simulink model "MSDRPrimaryLoop_LoadFollow"  (R2021b)
settings: Solver=VariableStepAuto  StartTime=0.0  StopTime=604900  MaxStep=1  MinStep=0.01  RelTol=1e-3
undefined symbols (not defined in the file): a_f, A_free_PHX, a_g, A_h_PHX, beta, beta_t, bubbleGeneratorArea, bubbleGeneratorDh, bubbleGeneratorElevation, bubbleGeneratorLength, bubbleGeneratorVolume, bubbleSaturationLevel, bubbleSeparatorArea, bubbleSeparatorDiameter, bubbleSeparatorDo, bubbleSeparatorLength, bubbleSeparatorSlope, bypassRatio, C0, coreFlowArea, coreFuelVolume, coreLowerPlenumArea, coreLowerPlenumHydraulicDiameter, coreLowerPlenumLength, coreLowerPlenumVolume, coreUpperPlenumArea, coreUpperPlenumHydraulicDiameter, coreUpperPlenumLength, coreUpperPlenumVolume, coreVolume, cpGraphite, dissolusionRatio, dMin, dScale, dsmConst, DXeG, Fiss_factor, fuelChannelHydrualicDiameter, fuelChannelLength, fuelDepositRatio, fuelFraction, fuelGraphiteArea, fuelGraphiteHeatTransferCoefficient, gamma0, gamma1, gamma2, generatorDsm, graphiteKDiff, graphiteUnitCellThickness, initialIodineConcentration, InitialXeMolarConcentration, InjectionRatio, injectionRatio, iodineDecayConstant, IodineDecayConstant, iodineYield, kGraphite, kScale, Lam, lam ... (+60)
libraries: fl_lib x268, nesl_utility x106, SimscapeFluids_lib x20, slpidlib x1
(part 12 of 12)

== system MSDRPrimaryLoop_LoadFollow/Reactor/CoreTH&Inerti/Core/CoreXenonCalc/InterphaseTranfser/Constitutive ==
  alpha : Inport
  PLoss : Inport  Port=2
  VolumeRate : Inport  Port=3
  Diam : Inport  Port=4
  Absolute Reference (TL) : fl_lib/Thermal Liquid/Elements/Absolute Reference (TL)
      settings: SourceProductBaseCode=SS
  DiffusivityScale : Subsystem  ReferencedSubsystem=DiffusivityScale
  Divide : Product  Inputs=**/
  Divide1 : Product  Inputs=*/
  KScale : Subsystem  ReferencedSubsystem=KScale
  PS-Simulink Converter : nesl_utility/PS-Simulink Converter  PhysicalDomain=network_engine_domain  SubClassName=ps_output  LeftPortType=input  RightPortType=output  PseudoPeriodic=off  Frequencies=[]  Unit=inherit  AffineConversion=off
      settings: SourceProductBaseCode=PW,SS
  PS-Simulink Converter2 : nesl_utility/PS-Simulink Converter  PhysicalDomain=network_engine_domain  SubClassName=ps_output  LeftPortType=input  RightPortType=output  PseudoPeriodic=off  Frequencies=[]  Unit=inherit  AffineConversion=off
      settings: SourceProductBaseCode=PW,SS
  Pressure & Temperature Sensor (TL) : fl_lib/Thermal Liquid/Sensors/Pressure & Temperature Sensor (TL)
      settings: SourceProductBaseCode=SS  InternalSimscapePortConfiguration="{\"Bottom\":[],\"Left\":[{\"id\":\"A\",\"label\":\"A\",\"type\":\"foundation.thermal_liquid.thermal_liquid\"}],\"Right\":[{\"id\":\"B\",\"label\":\"B\",\"type\":\"foundation.thermal_liquid.thermal_liquid\"},{\"id\":\"P\",\"label\":\"P\",\"type\":\"output\"},{\"id\":\"T\",\"label\":\"T\",\"type\":\"output\"}],\"Top\":[]}"
  RateToVelocity : Gain  Gain=1/CoreFlowArea
  Simscape Component : SimscapeComponentBlock  SourceFile=TL_FullSensor  ComponentPath=TL_FullSensor  ComponentVariants="[\"TL_FullSensor\"]"  ComponentVariantNames="[\"TL_FullSensor\"]"  ClassName=TL_FullSensor  SchemaVersion=1
      settings: CopyFcn=simscape.engine.sli.internal.componentblockcallback(gcbh,'COPY')  PreCopyFcn=simscape.engine.sli.internal.componentblockcallback(gcbh,'PRECOPY')  PreDeleteFcn=simscape.engine.sli.internal.componentblockcallback(gcbh,'PREDELETE')  InternalSimscapePortConfiguration="{\"Bottom\":[],\"Left\":[{\"id\":\"A\",\"label\":\"A\",\"type\":\"foundation.thermal_liquid.thermal_liquid\"}],\"Right\":[{\"id\":\"U\",\"label\":\"u\",\"type\":\"output\"},{\"id\":\"RHO\",\"label\":\"rho\",\"type\":\"output\"},{\"id\":\"CP\",\"label\":\"cp\",\"type\":\"output\"},{\"id\":\"NU\",\"label\":\"nu\",\"type\":\"output\"}],\"Top\":[]}"
      mask Type: Thermodynamic Properties Sensor (TL)
  Subsystem : Subsystem
      settings: PortSchema="{\"entries\":[{\"content\":{\"sides\":[{\"content\":{\"connectorIds\":[\"In1\",\"In2\",\"In3\"]},\"type\":\"ConnectorPlacement.EquallySpacedRectSide\",\"uuid\":\"97ac891d-0429-4bc8-a60c-b0f3d1709d12\"},{\"content\":{\"connectorIds\":[\"Out1\",\"Out2\"],\"side\":\"RIGHT\"},\"type\":\"ConnectorPlacement.EquallySpacedRectSide\",\"uuid\":\"927322a9-25fd-4042-b3db-749c2dfc8e8e\"},{\"content\":{\"connectorIds\":[\"In4\"],\"side\":\"TOP\"},\"type\":\"ConnectorPlacement.EquallySpacedRectSide\",\"uuid\":\"5b5a100b-866f-4829-ad8d-b4d6b97554c9\"},{\"content\":{\"connectorIds\":[\"RConn1\"],\"side\":\"BOTTOM\"},\"type\":\"ConnectorPlacement.EquallySpacedRectSide\",\"uuid\":\"36595118-997d-4e8e-8858-46ba20a030b3\"}]},\"type\":\"ConnectorPlacement.EquallySpacedConnector\",\"uuid\":\"6add3457-58ee-40cf-aa0f-ff6fc47a0098\"}],\"packageUris\":[\"http://schema.mathworks.com/mf0/Connector/R2020b\"],\"version\":\"1.0\"}"
  Ref : PMIOPort  Side=Left
  ul : Outport
  ug : Outport  Port=2
  K : Outport  Port=3
  Re : Outport  Port=4
  Sc : Outport  Port=5
  Diff : Outport  Port=6
  alphaC : Outport  Port=7
  dsm : Outport  Port=8
  f_m : Outport  Port=9
  wires:
  alpha/1 -> alphaC/1, Subsystem/4(alpha)
  VolumeRate/1 -> RateToVelocity/1
  RateToVelocity/1 -> ug/1, Subsystem/3(ul), ul/1, Divide/1
  Diam/1 -> Subsystem/2(Dh), Divide/2
  PS-Simulink Converter/1 -> Divide/3, Divide1/1
  PS-Simulink Converter2/1 -> DiffusivityScale/1, KScale/1
  DiffusivityScale/1 -> Divide1/2, Diff/1
  Divide1/1 -> Sc/1
  KScale/1 -> K/1
  Subsystem/2(dsm) -> dsm/1
  Divide/1 -> Re/1
  PLoss/1 -> Subsystem/1(PLoss)
  Subsystem/1(f_Combined) -> f_m/1
  connections:
  Pressure & Temperature Sensor (TL)/LConn1 -- Subsystem/RConn1 -- Simscape Component/LConn1 -- Ref/RConn1
  Simscape Component/RConn4 -- PS-Simulink Converter/LConn1
  Pressure & Temperature Sensor (TL)/RConn3 -- PS-Simulink Converter2/LConn1
  Pressure & Temperature Sensor (TL)/RConn1 -- Absolute Reference (TL)/LConn1

== system MSDRPrimaryLoop_LoadFollow/Reactor/CoreTH&Inerti/Core/CoreXenonCalc/InterphaseTranfser/GraphiteInterchangeModel ==
  CXef : Inport
  phi : Inport  Port=2
  Tempature : Inport  Port=3
  CXeg : Inport  Port=4
  dsm : Inport  Port=5
  GasRef : Inport  Port=6
  ul : Inport  Port=7
  Constant : Constant  Value=shapeFactor
  Constant1 : Constant  Value=graphiteKDiff
  DiffRateGas : Gain  Gain=FuelGraphiteArea
  DiffRateSalt : Gain  Gain=FuelGraphiteArea
  DiffusivityScale : Subsystem  ReferencedSubsystem=DiffusivityScale
  Gain3 : Gain  Gain=GraphitePorosity*GraphiteVolume
  GasDiffusivityScale : Subsystem
  GraphiteDiffusion : MATLAB Function  TreatAsAtomicUnit=on
  KScale : Subsystem  ReferencedSubsystem=KScale
  SimulationTime : Clock
  To Workspace : ToWorkspace  VariableName=C_face  SaveFormat=Timeseries  SampleTime=10000
  To Workspace1 : ToWorkspace  VariableName=C_Xef  SaveFormat=Timeseries  SampleTime=10000
  To Workspace2 : ToWorkspace  VariableName=C_Xeg  SaveFormat=Timeseries  SampleTime=10000
  Salt Diffusion Rate : Outport
  Xenon Mass In Graphite : Outport  Port=2
  Gas Diffusion Rate : Outport  Port=3
  wires:
  GraphiteDiffusion/3(xe_pvolave_conc) -> Gain3/1
  GraphiteDiffusion/1(fluxSalt) -> DiffRateSalt/1
  DiffRateSalt/1 -> Salt Diffusion Rate/1
  Gain3/1 -> Xenon Mass In Graphite/1
  phi/1 -> GraphiteDiffusion/4(phi)
  SimulationTime/1 -> GraphiteDiffusion/1(tnp1)
  Tempature/1 -> GasDiffusivityScale/1(T), KScale/1, DiffusivityScale/1
  KScale/1 -> GraphiteDiffusion/6(K)
  DiffusivityScale/1 -> GraphiteDiffusion/7(Df)
  GasDiffusivityScale/1(DiffGas) -> GraphiteDiffusion/8(Dg)
  CXeg/1 -> To Workspace2/1, GraphiteDiffusion/3(CXeg)
  GraphiteDiffusion/2(fluxGas) -> DiffRateGas/1
  DiffRateGas/1 -> Gas Diffusion Rate/1
  Constant/1 -> GraphiteDiffusion/10(shapeFactor)
  GasRef/1 -> GraphiteDiffusion/5(alpha)
  GraphiteDiffusion/4(C_face) -> To Workspace/1
  CXef/1 -> To Workspace1/1, GraphiteDiffusion/2(CXef)
  dsm/1 -> GraphiteDiffusion/9(d)
  ul/1 -> GraphiteDiffusion/11(ul)
  Constant1/1 -> GraphiteDiffusion/12(graphiteKD)

== system MSDRPrimaryLoop_LoadFollow/Reactor/CoreTH&Inerti/Core/CoreXenonCalc/Salt/InCoreGeneration ==
  NeutronFraction : Inport
  IodineSNumberDensity : Inport  Port=2
  T_f_ave : Inport  Port=3
  Add : Sum
  DecayXenonGenerationRate : Product
  DirectXeGenerationRate : Product
  DirectYield : Constant  Value=xe135Yield
  Molar/s : Product  Inputs=*/
  Na : Constant  Value=6.022e23
  NominalFissionRate : Constant  Value=ReactorPower/(200*1e6*1.602e-19)
  P1 : Product
  T2Rho : Fcn  Expr=3960 - 0.6724*u
  gain : Gain  Gain=iodineDecayConstant*CoreVolume*FuelFraction
  kg/s : Gain  Gain=0.135
  "XenonGenerationRate, [kg/s]" : Outport
  wires:
  NominalFissionRate/1 -> P1/1
  DirectYield/1 -> P1/2
  P1/1 -> DirectXeGenerationRate/2
  NeutronFraction/1 -> DirectXeGenerationRate/1
  IodineSNumberDensity/1 -> gain/1
  T_f_ave/1 -> T2Rho/1
  gain/1 -> DecayXenonGenerationRate/1
  T2Rho/1 -> DecayXenonGenerationRate/2
  DecayXenonGenerationRate/1 -> Add/1
  DirectXeGenerationRate/1 -> Add/2
  Add/1 -> Molar/s/1
  Na/1 -> Molar/s/2
  Molar/s/1 -> kg/s/1
  kg/s/1 -> "XenonGenerationRate, [kg/s]"/1

== system MSDRPrimaryLoop_LoadFollow/Reactor/CoreTH&Inerti/Core/CoreXenonCalc/Salt/Subsystem1 ==
  Gas : Inport
  Add1 : Sum  Inputs=+-
  Constant : Constant
  Subsystem : Subsystem  ReferencedSubsystem=GasToAlpha
  1-alpha : Outport
  wires:
  Gas/1 -> Subsystem/1
  Constant/1 -> Add1/1
  Subsystem/1 -> Add1/2
  Add1/1 -> 1-alpha/1

== system MSDRPrimaryLoop_LoadFollow/Reactor/CoreTH&Inerti/Core/Subsystem2/Subsystem2/If Action Subsystem ==
  GasIn : Inport
  AbsorbedOut : Inport  Port=2
  XeIn : Inport  Port=3
  Action Port : ActionPort  ActionPortLabel=if(u1 > 0)
  SolubilityModificationEqual : Subsystem  VariantControl=Equal
  GasOut : Outport
  XeOut : Outport  Port=2
  wires:
  SolubilityModificationEqual/2(GasOut) -> GasOut/1
  SolubilityModificationEqual/1(XeOut) -> XeOut/1
  XeIn/1 -> SolubilityModificationEqual/1(XeIn)
  AbsorbedOut/1 -> SolubilityModificationEqual/3(DissolvedGas)
  GasIn/1 -> SolubilityModificationEqual/2(CoreGas)

== system MSDRPrimaryLoop_LoadFollow/Reactor/CoreTH&Inerti/Core/Subsystem2/Subsystem2/If Action Subsystem1 ==
  GasIn : Inport
  AbsorbedOut : Inport  Port=2
  XeIn : Inport  Port=3
  Temperature : Inport  Port=4
  Action Port : ActionPort  ActionPortLabel=else
  SolubilityModificationPrescribed : Subsystem  VariantControl=Constant
      settings: PortSchema="{\"entries\":[{\"content\":{\"sides\":[{\"content\":{\"connectorIds\":[\"In1\",\"In2\",\"In3\"]},\"type\":\"ConnectorPlacement.EquallySpacedRectSide\",\"uuid\":\"65b34740-9d71-4003-bb50-ec967c02deea\"},{\"content\":{\"connectorIds\":[\"Out1\",\"Out2\"],\"side\":\"RIGHT\"},\"type\":\"ConnectorPlacement.EquallySpacedRectSide\",\"uuid\":\"1db9ab1c-1665-4743-8c97-35de06a35236\"},{\"content\":{\"connectorIds\":[\"In4\"],\"side\":\"TOP\"},\"type\":\"ConnectorPlacement.EquallySpacedRectSide\",\"uuid\":\"810fac02-fdbc-4f7b-bc70-c875a1a7376a\"}]},\"type\":\"ConnectorPlacement.EquallySpacedConnector\",\"uuid\":\"578127e1-d7fd-408e-a8bf-bcecd6d9e4eb\"}],\"packageUris\":[\"http://schema.mathworks.com/mf0/Connector/R2020b\"],\"version\":\"1.0\"}"
  GasOut : Outport
  XeOut : Outport  Port=2
  wires:
  SolubilityModificationPrescribed/2(GasOut) -> GasOut/1
  SolubilityModificationPrescribed/1(XeOut) -> XeOut/1
  XeIn/1 -> SolubilityModificationPrescribed/1(XeIn)
  AbsorbedOut/1 -> SolubilityModificationPrescribed/3(DissolvedGas)
  GasIn/1 -> SolubilityModificationPrescribed/2(CoreGas)
  Temperature/1 -> SolubilityModificationPrescribed/4(Temperature)

== system MSDRPrimaryLoop_LoadFollow/Reactor/CoreTH&Inerti/LowerPlenum/XenonCalc/InterphaseTranfser/Constitutive ==
  alpha : Inport
  PLoss : Inport  Port=2
  VolumeRate : Inport  Port=3
  Diam : Inport  Port=4
  Absolute Reference (TL) : fl_lib/Thermal Liquid/Elements/Absolute Reference (TL)
      settings: SourceProductBaseCode=SS
  DiffusivityScale : Subsystem  ReferencedSubsystem=DiffusivityScale
  Divide : Product  Inputs=**/
  Divide1 : Product  Inputs=*/
  KScale : Subsystem  ReferencedSubsystem=KScale
  PS-Simulink Converter : nesl_utility/PS-Simulink Converter  PhysicalDomain=network_engine_domain  SubClassName=ps_output  LeftPortType=input  RightPortType=output  PseudoPeriodic=off  Frequencies=[]  Unit=inherit  AffineConversion=off
      settings: SourceProductBaseCode=PW,SS
  PS-Simulink Converter2 : nesl_utility/PS-Simulink Converter  PhysicalDomain=network_engine_domain  SubClassName=ps_output  LeftPortType=input  RightPortType=output  PseudoPeriodic=off  Frequencies=[]  Unit=inherit  AffineConversion=off
      settings: SourceProductBaseCode=PW,SS
  Pressure & Temperature Sensor (TL) : fl_lib/Thermal Liquid/Sensors/Pressure & Temperature Sensor (TL)
      settings: SourceProductBaseCode=SS  InternalSimscapePortConfiguration="{\"Bottom\":[],\"Left\":[{\"id\":\"A\",\"label\":\"A\",\"type\":\"foundation.thermal_liquid.thermal_liquid\"}],\"Right\":[{\"id\":\"B\",\"label\":\"B\",\"type\":\"foundation.thermal_liquid.thermal_liquid\"},{\"id\":\"P\",\"label\":\"P\",\"type\":\"output\"},{\"id\":\"T\",\"label\":\"T\",\"type\":\"output\"}],\"Top\":[]}"
  RateToVelocity : Gain  Gain=1/Area
  Simscape Component : SimscapeComponentBlock  SourceFile=TL_FullSensor  ComponentPath=TL_FullSensor  ComponentVariants="[\"TL_FullSensor\"]"  ComponentVariantNames="[\"TL_FullSensor\"]"  ClassName=TL_FullSensor  SchemaVersion=1
      settings: CopyFcn=simscape.engine.sli.internal.componentblockcallback(gcbh,'COPY')  PreCopyFcn=simscape.engine.sli.internal.componentblockcallback(gcbh,'PRECOPY')  PreDeleteFcn=simscape.engine.sli.internal.componentblockcallback(gcbh,'PREDELETE')  InternalSimscapePortConfiguration="{\"Bottom\":[],\"Left\":[{\"id\":\"A\",\"label\":\"A\",\"type\":\"foundation.thermal_liquid.thermal_liquid\"}],\"Right\":[{\"id\":\"U\",\"label\":\"u\",\"type\":\"output\"},{\"id\":\"RHO\",\"label\":\"rho\",\"type\":\"output\"},{\"id\":\"CP\",\"label\":\"cp\",\"type\":\"output\"},{\"id\":\"NU\",\"label\":\"nu\",\"type\":\"output\"}],\"Top\":[]}"
      mask Type: Thermodynamic Properties Sensor (TL)
  dsmFun : Subsystem  ReferencedSubsystem=dsmFun
      settings: PortSchema="{\"entries\":[{\"content\":{\"sides\":[{\"content\":{\"connectorIds\":[\"In2\",\"In3\",\"In4\"]},\"type\":\"ConnectorPlacement.EquallySpacedRectSide\",\"uuid\":\"cd878d6d-d881-48a3-8bcf-2f6377bc2619\"},{\"content\":{\"connectorIds\":[\"Out1\",\"Out2\"],\"side\":\"RIGHT\"},\"type\":\"ConnectorPlacement.EquallySpacedRectSide\",\"uuid\":\"84ec48cd-6af4-419c-aaeb-7134212c3ae2\"},{\"content\":{\"connectorIds\":[\"In1\"],\"side\":\"TOP\"},\"type\":\"ConnectorPlacement.EquallySpacedRectSide\",\"uuid\":\"d836bcb8-c56c-40d6-b9ba-0790b759147b\"},{\"content\":{\"connectorIds\":[\"RConn1\"],\"side\":\"BOTTOM\"},\"type\":\"ConnectorPlacement.EquallySpacedRectSide\",\"uuid\":\"16763d39-53e3-4dc4-9c8a-2531c5df2d8d\"}]},\"type\":\"ConnectorPlacement.EquallySpacedConnector\",\"uuid\":\"ad3a93fd-9624-45a3-bd6b-21e42fcd018d\"}],\"packageUris\":[\"http://schema.mathworks.com/mf0/Connector/R2020b\"],\"version\":\"1.0\"}"
  Ref : PMIOPort  Side=Left
  ul : Outport
  ug : Outport  Port=2
  K : Outport  Port=3
  Re : Outport  Port=4
  Sc : Outport  Port=5
  Diff : Outport  Port=6
  alphaC : Outport  Port=7
  dsm : Outport  Port=8
  f_m : Outport  Port=9
  wires:
  alpha/1 -> dsmFun/1, alphaC/1
  VolumeRate/1 -> RateToVelocity/1
  RateToVelocity/1 -> ug/1, dsmFun/4, ul/1, Divide/1
  Diam/1 -> dsmFun/3, Divide/2
  PS-Simulink Converter/1 -> Divide/3, Divide1/1
  PS-Simulink Converter2/1 -> DiffusivityScale/1, KScale/1
  DiffusivityScale/1 -> Divide1/2, Diff/1
  Divide1/1 -> Sc/1
  KScale/1 -> K/1
  dsmFun/2 -> dsm/1
  Divide/1 -> Re/1
  PLoss/1 -> dsmFun/2
  dsmFun/1 -> f_m/1
  connections:
  Pressure & Temperature Sensor (TL)/LConn1 -- dsmFun/RConn1 -- Simscape Component/LConn1 -- Ref/RConn1
  Simscape Component/RConn4 -- PS-Simulink Converter/LConn1
  Pressure & Temperature Sensor (TL)/RConn3 -- PS-Simulink Converter2/LConn1
  Pressure & Temperature Sensor (TL)/RConn1 -- Absolute Reference (TL)/LConn1

== system MSDRPrimaryLoop_LoadFollow/Reactor/CoreTH&Inerti/LowerPlenum/XenonCalc/Salt/InPipeGeneration ==
  IodineSNumberDensity : Inport
  T_f_ave : Inport  Port=2
  DecayXenonGenerationRate : Product
  Molar/s : Product  Inputs=*/
  Na : Constant  Value=6.022e23
  T2Rho : Fcn  Expr=3960 - 0.6724*u
  gain : Gain  Gain=iodineDecayConstant*Volume
  kg/s : Gain  Gain=0.135
  "XenonGenerationRate, [kg/s]" : Outport
  wires:
  IodineSNumberDensity/1 -> gain/1
  T_f_ave/1 -> T2Rho/1
  gain/1 -> DecayXenonGenerationRate/1
  T2Rho/1 -> DecayXenonGenerationRate/2
  DecayXenonGenerationRate/1 -> Molar/s/1
  Na/1 -> Molar/s/2
  Molar/s/1 -> kg/s/1
  kg/s/1 -> "XenonGenerationRate, [kg/s]"/1

== system MSDRPrimaryLoop_LoadFollow/Reactor/CoreTH&Inerti/LowerPlenum/XenonCalc/Salt/Subsystem1 ==
  Gas : Inport
  Add1 : Sum  Inputs=+-
  Constant : Constant
  Subsystem : Subsystem  ReferencedSubsystem=GasToAlpha
  1-alpha : Outport
  wires:
  Gas/1 -> Subsystem/1
  Constant/1 -> Add1/1
  Subsystem/1 -> Add1/2
  Add1/1 -> 1-alpha/1

== system MSDRPrimaryLoop_LoadFollow/Reactor/CoreTH&Inerti/UpperPlenum/XenonCalc/InterphaseTranfser/Constitutive ==
  alpha : Inport
  PLoss : Inport  Port=2
  VolumeRate : Inport  Port=3
  Diam : Inport  Port=4
  Absolute Reference (TL) : fl_lib/Thermal Liquid/Elements/Absolute Reference (TL)
      settings: SourceProductBaseCode=SS
  DiffusivityScale : Subsystem  ReferencedSubsystem=DiffusivityScale
  Divide : Product  Inputs=**/
  Divide1 : Product  Inputs=*/
  KScale : Subsystem  ReferencedSubsystem=KScale
  PS-Simulink Converter : nesl_utility/PS-Simulink Converter  PhysicalDomain=network_engine_domain  SubClassName=ps_output  LeftPortType=input  RightPortType=output  PseudoPeriodic=off  Frequencies=[]  Unit=inherit  AffineConversion=off
      settings: SourceProductBaseCode=PW,SS
  PS-Simulink Converter2 : nesl_utility/PS-Simulink Converter  PhysicalDomain=network_engine_domain  SubClassName=ps_output  LeftPortType=input  RightPortType=output  PseudoPeriodic=off  Frequencies=[]  Unit=inherit  AffineConversion=off
      settings: SourceProductBaseCode=PW,SS
  Pressure & Temperature Sensor (TL) : fl_lib/Thermal Liquid/Sensors/Pressure & Temperature Sensor (TL)
      settings: SourceProductBaseCode=SS  InternalSimscapePortConfiguration="{\"Bottom\":[],\"Left\":[{\"id\":\"A\",\"label\":\"A\",\"type\":\"foundation.thermal_liquid.thermal_liquid\"}],\"Right\":[{\"id\":\"B\",\"label\":\"B\",\"type\":\"foundation.thermal_liquid.thermal_liquid\"},{\"id\":\"P\",\"label\":\"P\",\"type\":\"output\"},{\"id\":\"T\",\"label\":\"T\",\"type\":\"output\"}],\"Top\":[]}"
  RateToVelocity : Gain  Gain=1/Area
  Simscape Component : SimscapeComponentBlock  SourceFile=TL_FullSensor  ComponentPath=TL_FullSensor  ComponentVariants="[\"TL_FullSensor\"]"  ComponentVariantNames="[\"TL_FullSensor\"]"  ClassName=TL_FullSensor  SchemaVersion=1
      settings: CopyFcn=simscape.engine.sli.internal.componentblockcallback(gcbh,'COPY')  PreCopyFcn=simscape.engine.sli.internal.componentblockcallback(gcbh,'PRECOPY')  PreDeleteFcn=simscape.engine.sli.internal.componentblockcallback(gcbh,'PREDELETE')  InternalSimscapePortConfiguration="{\"Bottom\":[],\"Left\":[{\"id\":\"A\",\"label\":\"A\",\"type\":\"foundation.thermal_liquid.thermal_liquid\"}],\"Right\":[{\"id\":\"U\",\"label\":\"u\",\"type\":\"output\"},{\"id\":\"RHO\",\"label\":\"rho\",\"type\":\"output\"},{\"id\":\"CP\",\"label\":\"cp\",\"type\":\"output\"},{\"id\":\"NU\",\"label\":\"nu\",\"type\":\"output\"}],\"Top\":[]}"
      mask Type: Thermodynamic Properties Sensor (TL)
  dsmFun : Subsystem  ReferencedSubsystem=dsmFun
      settings: PortSchema="{\"entries\":[{\"content\":{\"sides\":[{\"content\":{\"connectorIds\":[\"In2\",\"In3\",\"In4\"]},\"type\":\"ConnectorPlacement.EquallySpacedRectSide\",\"uuid\":\"cd878d6d-d881-48a3-8bcf-2f6377bc2619\"},{\"content\":{\"connectorIds\":[\"Out1\",\"Out2\"],\"side\":\"RIGHT\"},\"type\":\"ConnectorPlacement.EquallySpacedRectSide\",\"uuid\":\"84ec48cd-6af4-419c-aaeb-7134212c3ae2\"},{\"content\":{\"connectorIds\":[\"In1\"],\"side\":\"TOP\"},\"type\":\"ConnectorPlacement.EquallySpacedRectSide\",\"uuid\":\"d836bcb8-c56c-40d6-b9ba-0790b759147b\"},{\"content\":{\"connectorIds\":[\"RConn1\"],\"side\":\"BOTTOM\"},\"type\":\"ConnectorPlacement.EquallySpacedRectSide\",\"uuid\":\"16763d39-53e3-4dc4-9c8a-2531c5df2d8d\"}]},\"type\":\"ConnectorPlacement.EquallySpacedConnector\",\"uuid\":\"ad3a93fd-9624-45a3-bd6b-21e42fcd018d\"}],\"packageUris\":[\"http://schema.mathworks.com/mf0/Connector/R2020b\"],\"version\":\"1.0\"}"
  Ref : PMIOPort  Side=Left
  ul : Outport
  ug : Outport  Port=2
  K : Outport  Port=3
  Re : Outport  Port=4
  Sc : Outport  Port=5
  Diff : Outport  Port=6
  alphaC : Outport  Port=7
  dsm : Outport  Port=8
  f_m : Outport  Port=9
  wires:
  alpha/1 -> alphaC/1, dsmFun/1
  VolumeRate/1 -> RateToVelocity/1
  RateToVelocity/1 -> ug/1, dsmFun/4, ul/1, Divide/1
  Diam/1 -> Divide/2, dsmFun/3
  PS-Simulink Converter/1 -> Divide/3, Divide1/1
  PS-Simulink Converter2/1 -> DiffusivityScale/1, KScale/1
  DiffusivityScale/1 -> Divide1/2, Diff/1
  Divide1/1 -> Sc/1
  KScale/1 -> K/1
  dsmFun/2 -> dsm/1
  Divide/1 -> Re/1
  dsmFun/1 -> f_m/1
  PLoss/1 -> dsmFun/2
  connections:
  Pressure & Temperature Sensor (TL)/LConn1 -- dsmFun/RConn1 -- Simscape Component/LConn1 -- Ref/RConn1
  Simscape Component/RConn4 -- PS-Simulink Converter/LConn1
  Pressure & Temperature Sensor (TL)/RConn3 -- PS-Simulink Converter2/LConn1
  Pressure & Temperature Sensor (TL)/RConn1 -- Absolute Reference (TL)/LConn1

== system MSDRPrimaryLoop_LoadFollow/Reactor/CoreTH&Inerti/UpperPlenum/XenonCalc/Salt/InPipeGeneration ==
  IodineSNumberDensity : Inport
  T_f_ave : Inport  Port=2
  DecayXenonGenerationRate : Product
  Molar/s : Product  Inputs=*/
  Na : Constant  Value=6.022e23
  T2Rho : Fcn  Expr=3960 - 0.6724*u
  gain : Gain  Gain=iodineDecayConstant*Volume
  kg/s : Gain  Gain=0.135
  "XenonGenerationRate, [kg/s]" : Outport
  wires:
  IodineSNumberDensity/1 -> gain/1
  gain/1 -> DecayXenonGenerationRate/1
  T_f_ave/1 -> T2Rho/1
  DecayXenonGenerationRate/1 -> Molar/s/1
  Na/1 -> Molar/s/2
  Molar/s/1 -> kg/s/1
  kg/s/1 -> "XenonGenerationRate, [kg/s]"/1
  T2Rho/1 -> DecayXenonGenerationRate/2

== system MSDRPrimaryLoop_LoadFollow/Reactor/CoreTH&Inerti/UpperPlenum/XenonCalc/Salt/Subsystem1 ==
  Gas : Inport
  Add1 : Sum  Inputs=+-
  Constant : Constant
  Subsystem : Subsystem  ReferencedSubsystem=GasToAlpha
  1-alpha : Outport
  wires:
  Gas/1 -> Subsystem/1
  Constant/1 -> Add1/1
  Subsystem/1 -> Add1/2
  Add1/1 -> 1-alpha/1

== system MSDRPrimaryLoop_LoadFollow/Reactor/CoreTH&Inerti/Core/CoreXenonCalc/InterphaseTranfser/Constitutive/Subsystem ==
  note: Include the form loss to averaged frictional factor as a rough estimate.
  PLoss : Inport
  Dh : Inport  Port=2
  ul : Inport  Port=3
  alpha : Inport  Port=4
  Absolute Reference (TL) : fl_lib/Thermal Liquid/Elements/Absolute Reference (TL)
      settings: SourceProductBaseCode=SS
  Constant : Constant  Value=dissolusionRatio
  Constant1 : Constant  Value=dMin
  Constant2 : Constant  Value=dScale
  Constant3 : Constant  Value=dsmConst
  Divide : Product  Inputs=**//
  Gain : Gain  Gain=2/CoreLength
  MATLAB Function1 : MATLAB Function  TreatAsAtomicUnit=on
  MATLAB Function2 : MATLAB Function  TreatAsAtomicUnit=on
  Math Function : Math  Operator=square  SaturateOnIntegerOverflow=on
  PS-Simulink Converter : nesl_utility/PS-Simulink Converter  PhysicalDomain=network_engine_domain  SubClassName=ps_output  LeftPortType=input  RightPortType=output  PseudoPeriodic=off  Frequencies=[]  Unit=inherit  AffineConversion=off
      settings: SourceProductBaseCode=PW,SS
  PS-Simulink Converter1 : nesl_utility/PS-Simulink Converter  PhysicalDomain=network_engine_domain  SubClassName=ps_output  LeftPortType=input  RightPortType=output  PseudoPeriodic=off  Frequencies=[]  Unit=inherit  AffineConversion=off
      settings: SourceProductBaseCode=PW,SS
  Pressure & Temperature Sensor (TL) : fl_lib/Thermal Liquid/Sensors/Pressure & Temperature Sensor (TL)
      settings: SourceProductBaseCode=SS  InternalSimscapePortConfiguration="{\"Bottom\":[],\"Left\":[{\"id\":\"A\",\"label\":\"A\",\"type\":\"foundation.thermal_liquid.thermal_liquid\"}],\"Right\":[{\"id\":\"B\",\"label\":\"B\",\"type\":\"foundation.thermal_liquid.thermal_liquid\"},{\"id\":\"P\",\"label\":\"P\",\"type\":\"output\"},{\"id\":\"T\",\"label\":\"T\",\"type\":\"output\"}],\"Top\":[]}"
  Simscape Component : SimscapeComponentBlock  SourceFile=TL_FullSensor  ComponentPath=TL_FullSensor  ComponentVariants="[\"TL_FullSensor\"]"  ComponentVariantNames="[\"TL_FullSensor\"]"  ClassName=TL_FullSensor  SchemaVersion=1
      settings: CopyFcn=simscape.engine.sli.internal.componentblockcallback(gcbh,'COPY')  PreCopyFcn=simscape.engine.sli.internal.componentblockcallback(gcbh,'PRECOPY')  PreDeleteFcn=simscape.engine.sli.internal.componentblockcallback(gcbh,'PREDELETE')  InternalSimscapePortConfiguration="{\"Bottom\":[],\"Left\":[{\"id\":\"A\",\"label\":\"A\",\"type\":\"foundation.thermal_liquid.thermal_liquid\"}],\"Right\":[{\"id\":\"U\",\"label\":\"u\",\"type\":\"output\"},{\"id\":\"RHO\",\"label\":\"rho\",\"type\":\"output\"},{\"id\":\"CP\",\"label\":\"cp\",\"type\":\"output\"},{\"id\":\"NU\",\"label\":\"nu\",\"type\":\"output\"}],\"Top\":[]}"
      mask Type: Thermodynamic Properties Sensor (TL)
  Terminator : Terminator
  Ref : PMIOPort  Side=Right
  f_Combined : Outport
  dsm : Outport  Port=2
  wires:
  Dh/1 -> Divide/2, MATLAB Function1/2(D)
  MATLAB Function2/1(sigma) -> MATLAB Function1/5(sigma)
  PS-Simulink Converter1/1 -> MATLAB Function2/1(T)
  ul/1 -> Math Function/1, MATLAB Function1/3(jl)
  PS-Simulink Converter/1 -> Divide/4, MATLAB Function1/4(rhol)
  PLoss/1 -> Gain/1
  Divide/1 -> f_Combined/1, MATLAB Function1/1(f)
  Gain/1 -> Divide/1
  Math Function/1 -> Divide/3
  alpha/1 -> MATLAB Function1/6(alpha)
  Constant/1 -> MATLAB Function1/7(alphaDissolve)
  Constant1/1 -> MATLAB Function1/8(dMin)
  Constant2/1 -> MATLAB Function1/9(scale)
  MATLAB Function1/1(dsm) -> dsm/1
  Constant3/1 -> Terminator/1
  connections:
  Simscape Component/RConn2 -- PS-Simulink Converter/LConn1
  Simscape Component/LConn1 -- Pressure & Temperature Sensor (TL)/LConn1 -- Ref/RConn1
  Pressure & Temperature Sensor (TL)/RConn3 -- PS-Simulink Converter1/LConn1
  Pressure & Temperature Sensor (TL)/RConn1 -- Absolute Reference (TL)/LConn1

== system MSDRPrimaryLoop_LoadFollow/Reactor/CoreTH&Inerti/Core/CoreXenonCalc/InterphaseTranfser/GraphiteInterchangeModel/GasDiffusivityScale ==
  T : Inport
  Constant : Constant  Value=1.5
  Divide : Product  Inputs=*/
  Divide1 : Product  Inputs=*/
  PReff : Constant  Value=1.013e5
  Power : Math  Operator=pow  SaturateOnIntegerOverflow=on
  Product : Product  Inputs=3
  TRef : Constant  Value=900
  XeReferenceDiff : Constant  Value=DXeG
  DiffGas : Outport
  wires:
  T/1 -> Divide/1
  TRef/1 -> Divide/2
  Divide/1 -> Power/1
  Constant/1 -> Power/2
  PReff/1 -> Divide1/1
  [coreAveragePressure] -> Divide1/2
  Power/1 -> Product/1
  Divide1/1 -> Product/2
  XeReferenceDiff/1 -> Product/3
  Product/1 -> DiffGas/1

== system MSDRPrimaryLoop_LoadFollow/Reactor/CoreTH&Inerti/Core/Subsystem2/Subsystem2/If Action Subsystem/SolubilityModificationEqual ==
  note: The idea is that when the dissolved gas comes back out, it is at the same salt concentration, assuming the nucleation process is fast, and it absorbed all xenon at the nucleation site but diffusion is not yet to kick in. As for the absorption into the old bubble, the saturation may be closer to 0, but never the less, the saturation level is already close to zero.
  XeIn : Inport
  CoreGas : Inport  Port=2
  DissolvedGas : Inport  Port=3
  Add : Sum
  Add1 : Sum
  AddedBackGas : Sum
  Constant : Constant
  Demux : Demux  Outputs=2
  Divide : Product  Inputs=**/
  Divide1 : Product  Inputs=*/
  Mux : Mux  Inputs=2
  XeOut : Outport
  GasOut : Outport  Port=2
  wires:
  CoreGas/1 -> AddedBackGas/1
  AddedBackGas/1 -> GasOut/1
  XeIn/1 -> Demux/1
  Mux/1 -> XeOut/1
  Constant/1 -> Add/2
  Add/1 -> Divide1/2, Divide/3
  Demux/1 -> Divide/1, Divide1/1
  Demux/2 -> Add1/1
  Divide/1 -> Add1/2
  Add1/1 -> Mux/2
  Divide1/1 -> Mux/1
  DissolvedGas/1 -> Add/1, Divide/2, AddedBackGas/2

== system MSDRPrimaryLoop_LoadFollow/Reactor/CoreTH&Inerti/Core/Subsystem2/Subsystem2/If Action Subsystem1/SolubilityModificationPrescribed ==
  note: The idea is that when the dissolved gas comes back out, it is saturated with xenon because of the super efficiency removal of micro bubbles. The gain factor is used to adjust the concentration of the bubbles to less than saturation.
  XeIn : Inport
  CoreGas : Inport  Port=2
  DissolvedGas : Inport  Port=3
  Temperature : Inport  Port=4
  Add : Sum
  Add1 : Sum
  AddedBackGas : Sum
  Constant : Constant
  Demux : Demux  Outputs=2
  Divide : Product  Inputs=**/
  Divide1 : Product  Inputs=*/
  Divide2 : Product  Inputs=*/
  Gain : Gain  Gain=bubbleSaturationLevel
  KScale : Subsystem  ReferencedSubsystem=KScale
  Mux : Mux  Inputs=2
  XeOut : Outport
  GasOut : Outport  Port=2
  wires:
  CoreGas/1 -> AddedBackGas/1
  DissolvedGas/1 -> Divide2/1, AddedBackGas/2
  AddedBackGas/1 -> GasOut/1
  XeIn/1 -> Demux/1
  Mux/1 -> XeOut/1
  Temperature/1 -> KScale/1
  KScale/1 -> Divide2/2
  Constant/1 -> Add/2
  Divide2/1 -> Gain/1
  Add/1 -> Divide1/2, Divide/3
  Demux/1 -> Divide/1, Divide1/1
  Demux/2 -> Add1/1
  Divide/1 -> Add1/2
  Add1/1 -> Mux/2
  Divide1/1 -> Mux/1
  Gain/1 -> Add/1, Divide/2

== matlab function MSDRPrimaryLoop_LoadFollow/pipeReactorToPump/XenonCalc/InterphaseTranfser/Transfer Term ==
  settings: updateMethod=DISCRETE
  data: GxS input; GxG input; volRate output; alpha input; ul input; ug input; K input; dsm input; k input
function volRate = Interpahse(GxS, GxG, alpha, ul, ug, K, dsm, k)

%Using GxS and GxG as variable is good for implementation to incorporate
%the initialization without divergence
volRate = 6*k/dsm*(K*GxG/ug - alpha/(1-alpha)*GxS/ul);

== matlab function MSDRPrimaryLoop_LoadFollow/Chemical Processing/ElevationPipe/XenonCalc/InterphaseTranfser1/Long Pipe Averaged Transfer Term ==
  settings: updateMethod=DISCRETE
  data: GxS input; GxG input; transferRate output; alpha input; ul input; ug input; K input; dsm input; k input; L input; Area input
function transferRate = Interpahse(GxS, GxG, alpha, ul, ug, K, dsm, k, L, Area)

%Using GxS and GxG as variable is good for implementation to incorporate
%the initialization without divergence

%Equation (3.21)
%volRate = 6*k/dsm*(K*GxG/ug - alpha/(1-alpha)*GxS/ul);

%The above equation could not be used for a long pipe section as GxS will
%be dropping considerably. 

%Here, we use Equation (3.26) in thesis, which is the difference bewteen
%GliIn and GliOut.


GxSInf = (GxS+GxG)./(1 + alpha./(1-alpha)./K*ug./ul);
GxSOut = (GxS-GxSInf).*exp(-6*k*L*alpha./(dsm.*ul.*(1-alpha))) + GxSInf;
dGxS = GxSOut-GxS;

transferRate = dGxS*Area;

== matlab function MSDRPrimaryLoop_LoadFollow/PHX/PHX Physical/XenonCalc1/InterphaseTranfser/Transfer Term ==
  settings: updateMethod=DISCRETE
  data: GxS input; GxG input; volRate output; alpha input; ul input; ug input; K input; dsm input; k input
function volRate = Interpahse(GxS, GxG, alpha, ul, ug, K, dsm, k)

%Using GxS and GxG as variable is good for implementation to incorporate
%the initialization without divergence
volRate = 6*k/dsm*(K*GxG/ug - alpha/(1-alpha)*GxS/ul);

== matlab function MSDRPrimaryLoop_LoadFollow/pipePHXToReactor/XenonCalc/InterphaseTranfser/Transfer Term ==
  settings: updateMethod=DISCRETE
  data: GxS input; GxG input; volRate output; alpha input; ul input; ug input; K input; dsm input; k input
function volRate = Interpahse(GxS, GxG, alpha, ul, ug, K, dsm, k)

%Using GxS and GxG as variable is good for implementation to incorporate
%the initialization without divergence
volRate = 6*k/dsm*(K*GxG/ug - alpha/(1-alpha)*GxS/ul);

== matlab function MSDRPrimaryLoop_LoadFollow/pipePumpToPHX/XenonCalc/InterphaseTranfser/Transfer Term ==
  settings: updateMethod=DISCRETE
  data: GxS input; GxG input; volRate output; alpha input; ul input; ug input; K input; dsm input; k input
function volRate = Interpahse(GxS, GxG, alpha, ul, ug, K, dsm, k)

%Using GxS and GxG as variable is good for implementation to incorporate
%the initialization without divergence
volRate = 6*k/dsm*(K*GxG/ug - alpha/(1-alpha)*GxS/ul);

== matlab function MSDRPrimaryLoop_LoadFollow/Chemical Processing/Bubble Separator/Subsystem/MATLAB Function ==
  data: alpha input; rho input; separatorEfficiency output; jl input; dP input; Do input; Lsp input; D input; k input; Re input; sigma input; mu input; dsm input
function separatorEfficiency = SepEff(alpha,rho,jl,dP,Do,Lsp,D,k,Re,sigma,mu,dsm)

if dP>0
    Dc = 1/3*D;
    deff = abs(sqrt(complex(dsm*sigma*D/mu/jl)*(1+tanh(100*alpha))));
    Dvoid = D*(D./deff)/k^2/real(Re).^0.4;
    effup = Do./(Do+0.0794*Dvoid)*tanh(4000*rho*real(jl)^2/dP);
    effdown = (1-effup)*0.3131*Do./(Do+0.0794*Dvoid)*tanh(0.075*Lsp/D)/(0.08*rho*real(jl)^2*Dc.^2./Do.^2./dP + 0.05);
    separatorEfficiency = min(effup + effdown,0.99);
else
    separatorEfficiency = 0;
end

== matlab function MSDRPrimaryLoop_LoadFollow/Reactor/CoreTH&Inerti/UpperPlenum/XenonCalc/InterphaseTranfser/Transfer Term ==
  settings: updateMethod=DISCRETE
  data: GxS input; GxG input; volRate output; alpha input; ul input; ug input; K input; dsm input; k input
function volRate = Interpahse(GxS, GxG, alpha, ul, ug, K, dsm, k)

%Using GxS and GxG as variable is good for implementation to incorporate
%the initialization without divergence
volRate = 6*k/dsm*(K*GxG/ug - alpha/(1-alpha)*GxS/ul);

== matlab function MSDRPrimaryLoop_LoadFollow/PHX/PHX Physical/XenonCalc1/InterphaseTranfser/k Calculation ==
  data: dsm output; Re input; k output; Sc input; Diff input; alpha input; dsm input; Diam input
function [dsm, k] = MassTransfer(Re, Sc, Diff, alpha, dsm, Diam)
    
    %Rough model at this moment by Kress.
    Sh = 0.34*Re^0.94*Sc^0.5*dsm/Diam;
    k = Sh/Diam*Diff;

end

== matlab function MSDRPrimaryLoop_LoadFollow/Reactor/CoreTH&Inerti/LowerPlenum/XenonCalc/InterphaseTranfser/Transfer Term ==
  settings: updateMethod=DISCRETE
  data: GxS input; GxG input; volRate output; alpha input; ul input; ug input; K input; dsm input; k input
function volRate = Interpahse(GxS, GxG, alpha, ul, ug, K, dsm, k)

%Using GxS and GxG as variable is good for implementation to incorporate
%the initialization without divergence
volRate = 6*k/dsm*(K*GxG/ug - alpha/(1-alpha)*GxS/ul);

== matlab function MSDRPrimaryLoop_LoadFollow/Reactor/CoreTH&Inerti/Core/CoreXenonCalc/InterphaseTranfser/Transfer Term ==
  settings: updateMethod=DISCRETE
  data: GxS input; GxG input; volRate output; alpha input; ul input; ug input; K input; dsm input; k input
function volRate = Interpahse(GxS, GxG, alpha, ul, ug, K, dsm, k)

%Using GxS and GxG as variable is good for implementation to incorporate
%the initialization without divergence
volRate = 6*k/dsm*(K*GxG/ug - alpha/(1-alpha)*GxS/ul);

== matlab function MSDRPrimaryLoop_LoadFollow/Chemical Processing/Bubble Generator/XenonCalc/InterphaseTranfser/Transfer Term ==
  settings: updateMethod=DISCRETE
  data: GxS input; GxG input; volRate output; alpha input; ul input; ug input; K input; dsm input; k input
function volRate = Interpahse(GxS, GxG, alpha, ul, ug, K, dsm, k)

%Using GxS and GxG as variable is good for implementation to incorporate
%the initialization without divergence
volRate = 6*k/dsm*(K*GxG/ug - alpha/(1-alpha)*GxS/ul);

== matlab function MSDRPrimaryLoop_LoadFollow/Chemical Processing/Bubble Separator/Subsystem/Constitutive/MATLAB Function2 ==
  data: T input; sigma output
function sigma = sigmaEquation(T)

T = T-273.15;
sigma = (235.5-0.09*T)*0.001; %Source from solubility in FLiBe by WATSON et al.

end

== matlab function MSDRPrimaryLoop_LoadFollow/Chemical Processing/PipeLine/XenonCalc/InterphaseTranfser/Long Pipe Averaged Transfer Term ==
  settings: updateMethod=DISCRETE
  data: GxS input; GxG input; transferRate output; alpha input; ul input; ug input; K input; dsm input; k input; L input; Area input
function transferRate = Interpahse(GxS, GxG, alpha, ul, ug, K, dsm, k, L, Area)

%Using GxS and GxG as variable is good for implementation to incorporate
%the initialization without divergence

%Equation (3.21)
%volRate = 6*k/dsm*(K*GxG/ug - alpha/(1-alpha)*GxS/ul);

%The above equation could not be used for a long pipe section as GxS will
%be dropping considerably. 

%Here, we use Equation (3.26) in thesis, which is the difference bewteen
%GliIn and GliOut.


GxSInf = (GxS+GxG)./(1 + alpha./(1-alpha)./K*ug./ul);
GxSOut = (GxS-GxSInf).*exp(-6*k*L*alpha./(dsm.*ul.*(1-alpha))) + GxSInf;
dGxS = GxSOut-GxS;

transferRate = dGxS*Area;

== matlab function MSDRPrimaryLoop_LoadFollow/Reactor/CoreTH&Inerti/Core/CoreXenonCalc/InterphaseTranfser/GraphiteInterchangeModel/GraphiteDiffusion ==
  settings: updateMethod=DISCRETE
  data: tnp1 input; CXef input; CXeg input; phi input; fluxSalt output; fluxGas output; alpha input; xe_pvolave_conc output; K input; Df input; Dg input; d input; shapeFactor input; C_face output; ul input; graphiteKD input
function [fluxSalt, fluxGas, xe_pvolave_conc, C_face] = xeMSREGraphite(tnp1, CXef,CXeg, phi, alpha, K, Df, Dg, d, shapeFactor, ul,graphiteKD)
%Solve diffusion into the graphite
    persistent tn
    persistent xegrid
    persistent rgrid
    persistent A
    persistent g

    porosity = 0.1;
    Dh = 0.0749; %MSDR unit flow cell.

    %It is expected that the regime is in laminar flow, the Kedl model used
    %a weird engineering correlation and gives a much larger
    %value for k. 
    kl = 3.66*Df/Dh;
    %Two layer model for overall mass transfer
    Rl = 1/kl;
    Rd = 0.2e-6/Df/sqrt(porosity);
    k = 1/(Rl + Rd);
  

    XeDecayConstant = 2.0916e-05;
    sigma_xe135 = 2.7e-18;

    R = 0.0277;
    dr = R/30;
    %Dk = 1.45e-8;
    Dk = graphiteKD; %A complicated topic, best left as a parameter.  See document.
    %Deff = 1.32e-8; %Taken from ORNL-4148 p35
    Deff = Dk*Dg/(Dk+Dg);
    
    ug = ul + 1e-3;
    dstar = real(sqrt(complex(Dg*d/ug)));
    
    shapeFactor = max(shapeFactor*exp(-5e-4/d)*porosity,4*k*real(sqrt(complex(d/Dg/ug))));


    Dg = shapeFactor * Dg;

    
    d = dstar;

    %Initialization of the persistent variables if the function is first
    %time being used
    if isempty(tn)
        tn = 0;
    end
    if isempty(rgrid)
        rgrid = linspace(0+dr/2,R-dr/2,30)';
    end
    if isempty(xegrid)
        xegrid = zeros(size(rgrid));
    end

    if isempty(g)
        g = zeros(size(rgrid));
        g(end) = (Deff/dr^2+Deff/2/dr)*2*k*dr/(2*porosity*Deff+K*k*dr)*CXef;
    end
    
    dt = tnp1 - tn;
    tn = tnp1;

    if dt <eps
        %Initialize to steady state condition if tnp1<=tn.
        tn = 0;
        phi0 = 0;
        phi = phi0;
        termp1 = Deff/dr^2*ones(length(rgrid)-1,1)+Deff/2/dr./rgrid(1:end-1);
        termm1 = Deff/dr^2*ones(length(rgrid)-1,1)-Deff/2/dr./rgrid(2:end);
        termdiag = -(2*Deff/dr^2+XeDecayConstant+phi*sigma_xe135)*ones(size(rgrid));
        lumpedDemominator = Dg*alpha*dr + 2*Deff*d*porosity + K*d*dr*k - K*alpha*d*dr*k;
        frontFactorCn = (2*Deff*d*porosity - Dg*alpha*dr - K*d*dr*k + K*alpha*d*dr*k)/lumpedDemominator;
        %reference no alpha, cn , (2*porosity*Deff-K*k*dr)/(2*porosity*Deff+K*k*dr)
        termdiag(end) = termdiag(end) + (Deff/dr^2+Deff/2/dr./rgrid(end))*frontFactorCn;
        A = diag(termp1,1)+diag(termm1,-1)+diag(termdiag);
        %reference no alpha, g, 2*k*dr/(2*porosity*Deff+K*k*dr)*CXef
        frontFactorBc = (2*Dg*alpha*CXeg*dr + 2*CXef*d*dr*k - 2*alpha*CXef*d*dr*k)/lumpedDemominator;
        g(end) = (Deff/dr^2+Deff/2/dr./rgrid(end))*frontFactorBc;

        xegrid = -A\g;
        %Reference no alpha, (2*porosity*Deff-K*k*dr)/(2*porosity*Deff+K*k*dr)*xegrid(end) + 2*k*dr/(2*porosity*Deff+K*k*dr)*CXef
        C_ghost = frontFactorBc + frontFactorCn*xegrid(end);
        C_face = (xegrid(end) + C_ghost)/2;

        fluxSalt = k*(K*C_face-CXef)*(1-alpha);
        fluxGas = alpha*Dg/d*(C_face-CXeg);
        
        %Calculate phase volume averaged concentration
        xe_pvolave_conc = sum(((rgrid+dr/2).^2-(rgrid-dr/2).^2).*xegrid)/R^2;


    else
        %Backward Euler time advancement scheme
        I = diag(ones(size(rgrid)));
        
        %Update time-dependent matrix
        termp1 = Deff/dr^2*ones(length(rgrid)-1,1)+Deff/2/dr./rgrid(1:end-1);
        termm1 = Deff/dr^2*ones(length(rgrid)-1,1)-Deff/2/dr./rgrid(2:end);
        termdiag = -(2*Deff/dr^2+XeDecayConstant+phi*sigma_xe135)*ones(size(rgrid));
        lumpedDemominator = Dg*alpha*dr + 2*Deff*d*porosity + K*d*dr*k - K*alpha*d*dr*k;
        frontFactorCn = (2*Deff*d*porosity - Dg*alpha*dr - K*d*dr*k + K*alpha*d*dr*k)/lumpedDemominator;
        %reference no alpha, cn , (2*porosity*Deff-K*k*dr)/(2*porosity*Deff+K*k*dr)
        termdiag(end) = termdiag(end) + (Deff/dr^2+Deff/2/dr./rgrid(end))*frontFactorCn;
        A = diag(termp1,1)+diag(termm1,-1)+diag(termdiag);
        %reference no alpha, g, 2*k*dr/(2*porosity*Deff+K*k*dr)*CXef
        frontFactorBc = (2*Dg*alpha*CXeg*dr + 2*CXef*d*dr*k - 2*alpha*CXef*d*dr*k)/lumpedDemominator;
        g(end) = (Deff/dr^2+Deff/2/dr./rgrid(end))*frontFactorBc;
        
        %Solve for new xenon concentration profile
        xegrid = (I-A*dt)\(g*dt+xegrid);
        
        %Calculate xenon flux in at the boundary
        C_ghost = frontFactorBc + frontFactorCn*xegrid(end);
        C_face = (xegrid(end) + C_ghost)/2;

        fluxSalt = k*(K*C_face-CXef)*(1-alpha);
        fluxGas = alpha*Dg/d*(C_face-CXeg);
        
        %Calculate phase volume averaged concentration
        xe_pvolave_conc = sum(((rgrid+dr/2).^2-(rgrid-dr/2).^2).*xegrid)/R^2;

    end

== matlab function MSDRPrimaryLoop_LoadFollow/Pump/PumpIdeal/XenonCalcPump/InterphaseTranfser/Transfer Term ==
  settings: updateMethod=DISCRETE
  data: CxS input; CxG input; volRate output; alpha input; K input; dsm input; k input
function volRate = InterpahseSimple(CxS, CxG, alpha, K, dsm, k)

%Using GxS and GxG as variable is good for implementation to incorporate
%the initialization without divergence
volRate = 6*k*alpha/dsm*(K*CxG - CxS);

== matlab function MSDRPrimaryLoop_LoadFollow/Reactor/CoreTH&Inerti/Core/CoreXenonCalc/InterphaseTranfser/Constitutive/Subsystem/MATLAB Function1 ==
  settings: updateMethod=DISCRETE
  data: f input; D input; jl input; rhol input; sigma input; dsm output; alpha input; alphaDissolve input; dMin input; scale input
function dsm = dsmTurbulent(f,D,jl,rhol,sigma,alpha,alphaDissolve,dMin,scale)

%alphaDissolve = max(eps,alphaDissolve);
dissipation = jl^3/2/D*abs(f);
dsm = scale*0.725/(rhol/sigma)^0.6/dissipation^0.4;
x = -atanh(2*dMin/dsm-1);
%dsm = max(dsm*(0.5 + 0.5*tanh(alpha*250-x))*(alpha./(alphaDissolve+alpha)).^(1/3),1e-5);
dsm = max(dsm*(0.5 + 0.5*tanh(alpha*100-x))*(alpha./(alphaDissolve+alpha)).^(1/3),1e-5);
%dsm = min(dsm,dMin*(1+alpha.^2))
dsm = min(dsm,D);

end

== matlab function MSDRPrimaryLoop_LoadFollow/Reactor/CoreTH&Inerti/Core/CoreXenonCalc/InterphaseTranfser/Constitutive/Subsystem/MATLAB Function2 ==
  data: T input; sigma output
function sigma = sigmaEquation(T)

T = T-273.15;
sigma = (235.5-0.09*T)*0.001; %Source from solubility in FLiBe by WATSON et al.

end

== matlab function MSDRPrimaryLoop_LoadFollow/PHX/PHX Ideal/XenonCalc/InterphaseTranfser/Transfer Term ==
  settings: updateMethod=DISCRETE
  data: GxS input; GxG input; volRate output; alpha input; ul input; ug input; K input; dsm input; k input
function volRate = Interpahse(GxS, GxG, alpha, ul, ug, K, dsm, k)

%Using GxS and GxG as variable is good for implementation to incorporate
%the initialization without divergence
volRate = 6*k/dsm*(K*GxG/ug - alpha/(1-alpha)*GxS/ul);
